simulink model "aircraft_sil"  (R2024a)
settings: Solver=ode45  StartTime=0.0  StopTime=2000  FixedStep=0.001  RelTol=1e-3
settings Model: PacingRate=100  Creator=ADMIN  LastModifiedBy=ADMIN

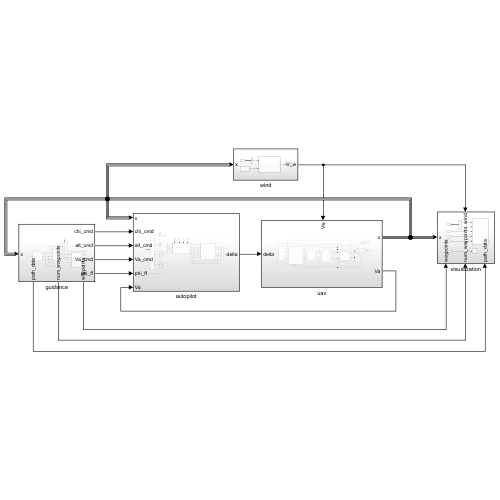
[thumbnail: Simulink's stored preview of the top-level diagram]
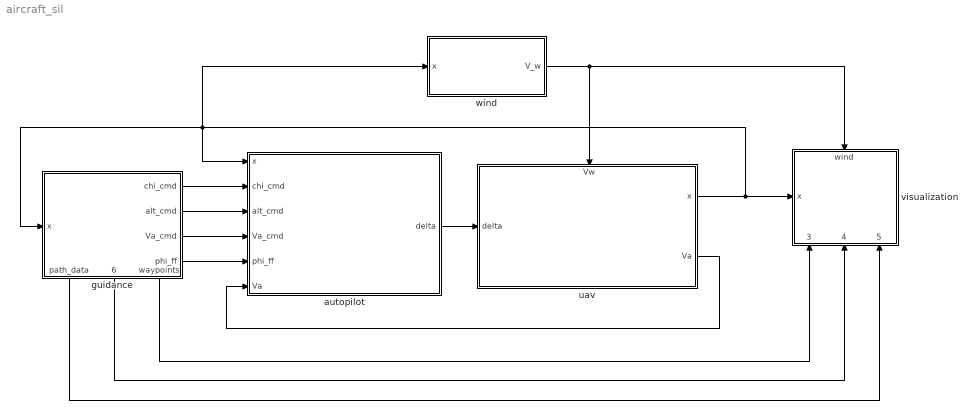
== system aircraft_sil ==
  "autopilot " : Subsystem
  guidance : Subsystem
      settings: PortSchema="{\"entries\":[{\"content\":{\"sides\":[{\"content\":{\"connectorIds\":[\"In1\"]},\"type\":\"ConnectorPlacement.EquallySpacedRectSide\",\"uuid\":\"7fb118f2-0b04-48cb-ae03-a27655c87a81\"},{\"content\":{\"connectorIds\":[\"Out1\",\"Out2\",\"Out3\",\"Out4\"],\"side\":\"RIGHT\"},\"type\":\"ConnectorPlacement.EquallySpacedRectSide\",\"uuid\":\"d962d9a4-ae5c-41e4-a82c-02c820f08147\"},{\"content\":{\"side\":\"TOP\"},\"type\":\"ConnectorPlacement.EquallySpacedRectSide\",\"uuid\":\"7cbabbb1-f237-4845-8a04-8eadc07c3469\"},{\"content\":{\"connectorIds\":[\"Out5\",\"Out6\",\"Out7\"],\"side\":\"BOTTOM\"},\"type\":\"ConnectorPlacement.EquallySpacedRectSide\",\"uuid\":\"34cfda24-2f18-4e48-95bb-4ae1da1686ef\"}]},\"type\":\"ConnectorPlacement.EquallySpacedConnector\",\"uuid\":\"2c187929-5ea7-462b-8474-1f36e513e0be\"}],\"packageUris\":[\"http://schema.mathworks.com/mf0/Connector/R2020b\"],\"version\":\"1.0\"}"
  "uav " : Subsystem
      settings: PortSchema="{\"entries\":[{\"content\":{\"sides\":[{\"content\":{\"connectorIds\":[\"In1\"]},\"type\":\"ConnectorPlacement.EquallySpacedRectSide\",\"uuid\":\"a7b46c76-63bb-4654-bcb2-91627cecb901\"},{\"content\":{\"connectorIds\":[\"Out1\",\"Out2\"],\"side\":\"RIGHT\"},\"type\":\"ConnectorPlacement.EquallySpacedRectSide\",\"uuid\":\"e45597e5-281a-43ae-9b8f-01f809ae90a8\"},{\"content\":{\"connectorIds\":[\"In2\"],\"side\":\"TOP\"},\"type\":\"ConnectorPlacement.EquallySpacedRectSide\",\"uuid\":\"e4f93d17-0834-49b6-953c-d959a9d487bc\"}]},\"type\":\"ConnectorPlacement.EquallySpacedConnector\",\"uuid\":\"aee35d44-0504-4876-b308-b0d63ae44a1f\"}],\"packageUris\":[\"http://schema.mathworks.com/mf0/Connector/R2020b\"],\"version\":\"1.0\"}"
  visualization : Subsystem
      settings: PortSchema="{\"entries\":[{\"content\":{\"sides\":[{\"content\":{\"connectorIds\":[\"In1\"]},\"type\":\"ConnectorPlacement.EquallySpacedRectSide\",\"uuid\":\"3ca85e6b-5690-4cee-b297-0410b8eb8b03\"},{\"content\":{\"side\":\"RIGHT\"},\"type\":\"ConnectorPlacement.EquallySpacedRectSide\",\"uuid\":\"b077d845-b4f0-4046-b1ae-a0ce879f315b\"},{\"content\":{\"connectorIds\":[\"In2\"],\"side\":\"TOP\"},\"type\":\"ConnectorPlacement.EquallySpacedRectSide\",\"uuid\":\"5282982d-07cb-4dd6-a7f3-d3fc714f27f8\"},{\"content\":{\"connectorIds\":[\"In3\",\"In4\",\"In5\"],\"side\":\"BOTTOM\"},\"type\":\"ConnectorPlacement.EquallySpacedRectSide\",\"uuid\":\"bf9b25fd-1836-4065-b749-44a2e35219bb\"}]},\"type\":\"ConnectorPlacement.EquallySpacedConnector\",\"uuid\":\"6eccf57b-fb72-419b-a501-32d6f52412a8\"}],\"packageUris\":[\"http://schema.mathworks.com/mf0/Connector/R2020b\"],\"version\":\"1.0\"}"
  wind : Subsystem
  wires:
  wind/1(V_w) -> visualization/2(wind), "uav "/2(Vw)
  "uav "/1(x) -> "autopilot "/1(x), guidance/1(x), wind/1(x), visualization/1(x)
  "autopilot "/1(delta) -> "uav "/1(delta)
  guidance/1(chi_cmd) -> "autopilot "/2(chi_cmd)
  guidance/2(alt_cmd) -> "autopilot "/3(alt_cmd)
  "uav "/2(Va) -> "autopilot "/6(Va)
  guidance/3(Va_cmd) -> "autopilot "/4(Va_cmd)
  guidance/4(phi_ff) -> "autopilot "/5(phi_ff)
  guidance/7(waypoints) -> visualization/3(waypoints)
  guidance/6(num_waypoints) -> visualization/4(num_waypoints)
  guidance/5(path_data) -> visualization/5(path_data)

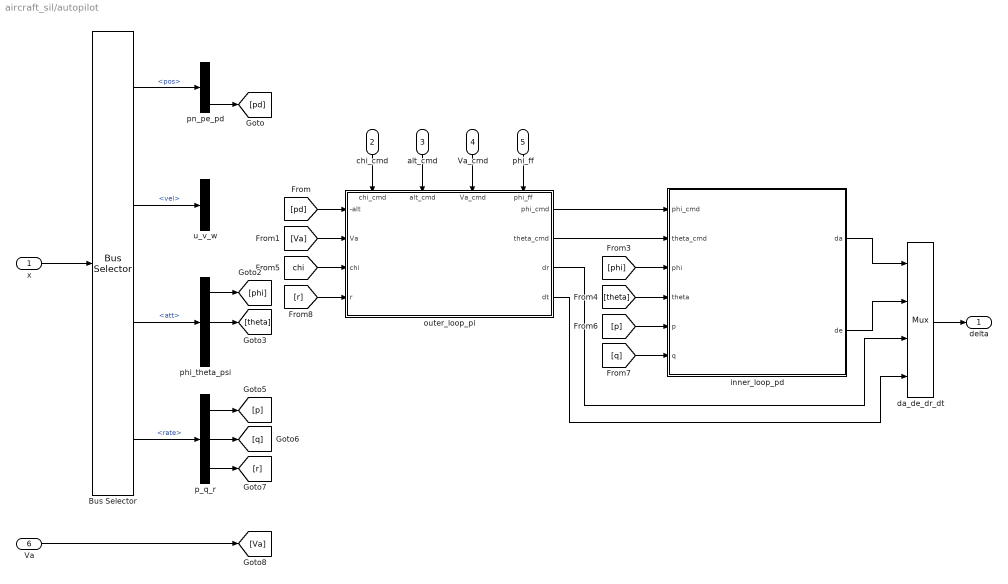
== system aircraft_sil/autopilot  ==
  x : Inport
  chi_cmd : Inport  Port=2
  alt_cmd : Inport  Port=3
  Va_cmd : Inport  Port=4
  phi_ff : Inport  Port=5
  Va : Inport  Port=6
  Bus Selector : BusSelector  OutputSignals=pos,vel,att,rate
  da_de_dr_dt : Mux
  inner_loop_pd : Subsystem
  outer_loop_pi : Subsystem
      settings: PortSchema="{\"entries\":[{\"content\":{\"sides\":[{\"content\":{\"connectorIds\":[\"In1\",\"In2\",\"In3\",\"In4\"]},\"type\":\"ConnectorPlacement.EquallySpacedRectSide\",\"uuid\":\"f8b93ce5-1209-4743-a4f6-40947377afa0\"},{\"content\":{\"connectorIds\":[\"Out1\",\"Out2\",\"Out3\",\"Out4\"],\"side\":\"RIGHT\"},\"type\":\"ConnectorPlacement.EquallySpacedRectSide\",\"uuid\":\"38b86da4-8ea0-4db2-a7be-1fc292de95ff\"},{\"content\":{\"connectorIds\":[\"In5\",\"In6\",\"In7\",\"In8\"],\"side\":\"TOP\"},\"type\":\"ConnectorPlacement.EquallySpacedRectSide\",\"uuid\":\"879dde49-1a12-4f2d-a7d9-4a8a8e5f8381\"}]},\"type\":\"ConnectorPlacement.EquallySpacedConnector\",\"uuid\":\"28f217f5-b437-4f7c-874d-3ab28b03532d\"}],\"packageUris\":[\"http://schema.mathworks.com/mf0/Connector/R2020b\"],\"version\":\"1.0\"}"
  p_q_r : Demux  Outputs=3
  phi_theta_psi : Demux  Outputs=3
  pn_pe_pd : Demux  Outputs=3
  u_v_w : Demux  Outputs=3
  delta : Outport
  wires:
  da_de_dr_dt/1 -> delta/1
  Bus Selector/3 -> phi_theta_psi/1  "<att>"
  Bus Selector/4 -> p_q_r/1  "<rate>"
  Bus Selector/1 -> pn_pe_pd/1  "<pos>"
  Bus Selector/2 -> u_v_w/1  "<vel>"
  inner_loop_pd/1(da) -> da_de_dr_dt/1
  inner_loop_pd/2(de) -> da_de_dr_dt/2
  outer_loop_pi/1(phi_cmd) -> inner_loop_pd/1(phi_cmd)
  outer_loop_pi/2(theta_cmd) -> inner_loop_pd/2(theta_cmd)
  outer_loop_pi/3(dr) -> da_de_dr_dt/3
  outer_loop_pi/4(dt) -> da_de_dr_dt/4
  pn_pe_pd/3 -> [pd]
  [pd] -> outer_loop_pi/1(-alt)
  [Va] -> outer_loop_pi/2(Va)
  phi_theta_psi/1 -> [phi]
  [phi] -> inner_loop_pd/3(phi)
  phi_theta_psi/2 -> [theta]
  [theta] -> inner_loop_pd/4(theta)
  [chi] -> outer_loop_pi/3(chi)
  p_q_r/1 -> [p]
  p_q_r/2 -> [q]
  [p] -> inner_loop_pd/5(p)
  [q] -> inner_loop_pd/6(q)
  p_q_r/3 -> [r]
  [r] -> outer_loop_pi/4(r)
  chi_cmd/1 -> outer_loop_pi/5(chi_cmd)
  alt_cmd/1 -> outer_loop_pi/6(alt_cmd)
  x/1 -> Bus Selector/1
  Va/1 -> [Va]
  Va_cmd/1 -> outer_loop_pi/7(Va_cmd)
  phi_ff/1 -> outer_loop_pi/8(phi_ff)

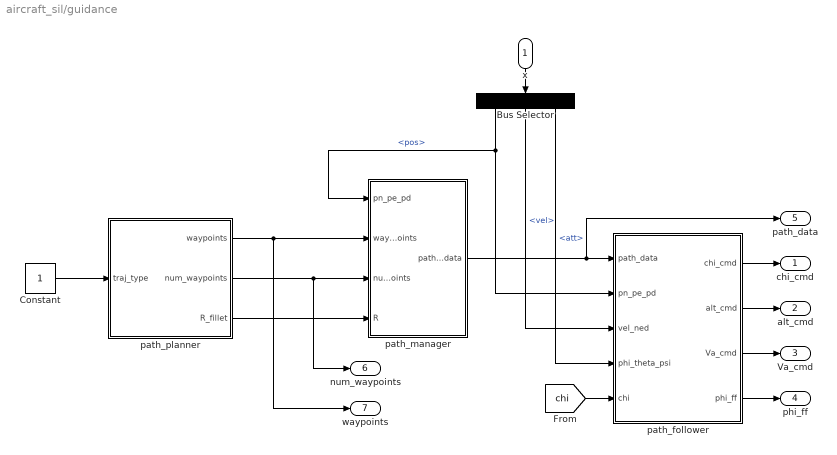
== system aircraft_sil/guidance ==
  x : Inport
  Bus Selector : BusSelector  OutputSignals=pos,vel,att
  Constant : Constant
  path_follower : MATLAB Function  TreatAsAtomicUnit=on
  path_manager : MATLAB Function  TreatAsAtomicUnit=on
  path_planner : MATLAB Function  TreatAsAtomicUnit=on
  chi_cmd : Outport
  alt_cmd : Outport  Port=2
  Va_cmd : Outport  Port=3
  phi_ff : Outport  Port=4
  path_data : Outport  Port=5
  num_waypoints : Outport  Port=6
  waypoints : Outport  Port=7
  wires:
  x/1 -> Bus Selector/1
  Bus Selector/1 -> path_manager/1(pn_pe_pd), path_follower/2(pn_pe_pd)  "<pos>"
  path_manager/1(path_data) -> path_data/1, path_follower/1(path_data)
  path_follower/1(chi_cmd) -> chi_cmd/1
  path_follower/2(alt_cmd) -> alt_cmd/1
  path_follower/3(Va_cmd) -> Va_cmd/1
  path_follower/4(phi_ff) -> phi_ff/1
  Bus Selector/2 -> path_follower/3(vel_ned)  "<vel>"
  Bus Selector/3 -> path_follower/4(phi_theta_psi)  "<att>"
  [chi] -> path_follower/5(chi)
  path_planner/1(waypoints) -> waypoints/1, path_manager/2(waypoints)
  path_planner/2(num_waypoints) -> num_waypoints/1, path_manager/3(num_waypoints)
  path_planner/3(R_fillet) -> path_manager/4(R)
  Constant/1 -> path_planner/1(traj_type)

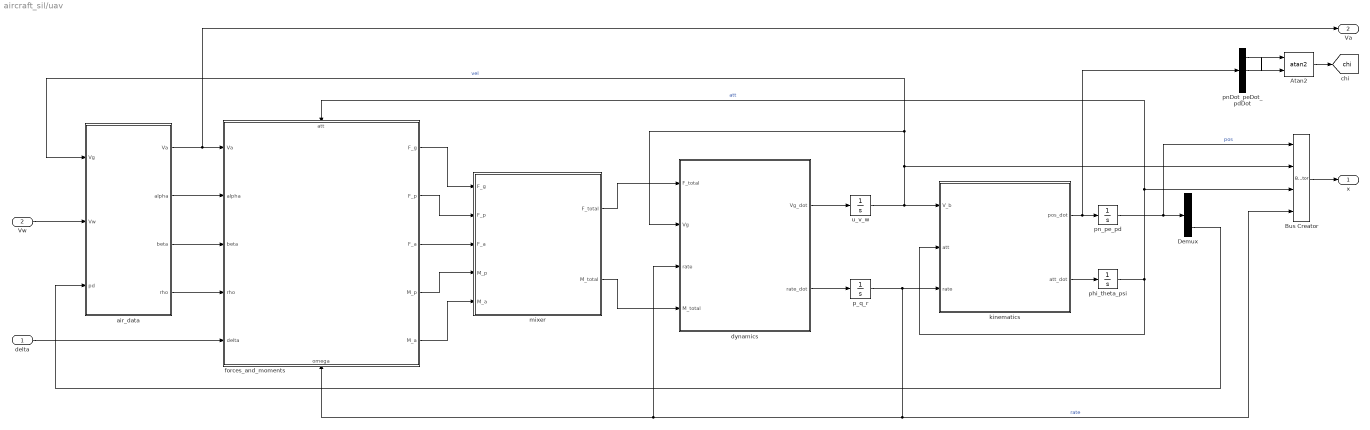
== system aircraft_sil/uav  ==
  delta : Inport
  Vw : Inport  Port=2
  Atan2 : Trigonometry  Operator=atan2
  Bus Creator : BusCreator  Inputs=4
  Demux : Demux  Outputs=3
  air_data : MATLAB Function  TreatAsAtomicUnit=on
  dynamics : Subsystem
  forces_and_moments : Subsystem
      settings: PortSchema="{\"entries\":[{\"content\":{\"sides\":[{\"content\":{\"connectorIds\":[\"In1\",\"In2\",\"In3\",\"In4\",\"In5\"]},\"type\":\"ConnectorPlacement.EquallySpacedRectSide\",\"uuid\":\"faed5ae1-1da7-4bdb-9f91-d07bb241893e\"},{\"content\":{\"connectorIds\":[\"Out1\",\"Out2\",\"Out3\",\"Out4\",\"Out5\"],\"side\":\"RIGHT\"},\"type\":\"ConnectorPlacement.EquallySpacedRectSide\",\"uuid\":\"3869cb38-1eed-4d47-9855-45677924a456\"},{\"content\":{\"connectorIds\":[\"In6\"],\"side\":\"TOP\"},\"type\":\"ConnectorPlacement.EquallySpacedRectSide\",\"uuid\":\"bdf63fef-403e-488a-a985-bca31845462f\"},{\"content\":{\"connectorIds\":[\"In7\"],\"side\":\"BOTTOM\"},\"type\":\"ConnectorPlacement.EquallySpacedRectSide\",\"uuid\":\"22a16173-6ad3-41e9-b567-c24186f01d1d\"}]},\"type\":\"ConnectorPlacement.EquallySpacedConnector\",\"uuid\":\"20fa0166-ef5c-40dd-8a30-826f9f2a65f7\"}],\"packageUris\":[\"http://schema.mathworks.com/mf0/Connector/R2020b\"],\"version\":\"1.0\"}"
  kinematics : Subsystem
  mixer : MATLAB Function  TreatAsAtomicUnit=on
  p_q_r : Integrator  InitialCondition=[0; 0; 0]
  phi_theta_psi : Integrator  InitialCondition=[0; 0.14622; 0]
  pnDot_peDot_pdDot : Demux  Outputs=3
  pn_pe_pd : Integrator  InitialCondition=[0; 0; -100]
  u_v_w : Integrator  InitialCondition=[15; 0; 3.3029]
  x : Outport
  Va : Outport  Port=2
  tag scope: chi=global
  wires:
  p_q_r/1 -> Bus Creator/4, dynamics/3(rate), forces_and_moments/7(omega), kinematics/3(rate)  "rate"
  kinematics/2(att_dot) -> phi_theta_psi/1
  u_v_w/1 -> kinematics/1(V_b), Bus Creator/2, air_data/1(Vg), dynamics/2(Vg)  "vel"
  pn_pe_pd/1 -> Bus Creator/1, Demux/1  "pos"
  dynamics/1(Vg_dot) -> u_v_w/1
  air_data/1(Va) -> Va/1, forces_and_moments/1(Va)
  phi_theta_psi/1 -> Bus Creator/3, forces_and_moments/6(att), kinematics/2(att)  "att"
  forces_and_moments/2(F_p) -> mixer/2(F_p)
  kinematics/1(pos_dot) -> pnDot_peDot_pdDot/1, pn_pe_pd/1
  forces_and_moments/3(F_a) -> mixer/3(F_a)
  Bus Creator/1 -> x/1
  mixer/1(F_total) -> dynamics/1(F_total)
  mixer/2(M_total) -> dynamics/4(M_total)
  Vw/1 -> air_data/2(Vw)
  air_data/2(alpha) -> forces_and_moments/2(alpha)
  air_data/3(beta) -> forces_and_moments/3(beta)
  forces_and_moments/1(F_g) -> mixer/1(F_g)
  forces_and_moments/4(M_p) -> mixer/4(M_p)
  air_data/4(rho) -> forces_and_moments/4(rho)
  forces_and_moments/5(M_a) -> mixer/5(M_a)
  Demux/3 -> air_data/3(pd)
  dynamics/2(rate_dot) -> p_q_r/1
  delta/1 -> forces_and_moments/5(delta)
  pnDot_peDot_pdDot/2 -> Atan2/1
  pnDot_peDot_pdDot/1 -> Atan2/2
  Atan2/1 -> [chi]

== system aircraft_sil/visualization ==
  x : Inport
  wind : Inport  Port=2
  waypoints : Inport  Port=3
  num_waypoints : Inport  Port=4
  path_data : Inport  Port=5
  Bus Selector : BusSelector  OutputSignals=pos,att
  MATLAB Function : MATLAB Function  TreatAsAtomicUnit=on
  wind_visualization : Scope
  wires:
  x/1 -> Bus Selector/1
  Bus Selector/1 -> MATLAB Function/1(pn_pe_pd)  "<pos>"
  Bus Selector/2 -> MATLAB Function/2(phi_theta_psi)  "<att>"
  wind/1 -> wind_visualization/1
  num_waypoints/1 -> MATLAB Function/4(num_waypoints)
  waypoints/1 -> MATLAB Function/3(waypoints)
  path_data/1 -> MATLAB Function/5(path_data)

== system aircraft_sil/wind ==
  x : Inport
  Bus Selector : BusSelector  OutputSignals=att
  Constant : Constant  Value=[0; 0; 0]
  MATLAB Function : MATLAB Function  TreatAsAtomicUnit=on
  V_w : Outport
  wires:
  x/1 -> Bus Selector/1
  Bus Selector/1 -> MATLAB Function/1(att)  "<att>"
  Constant/1 -> MATLAB Function/2(Vw_inertial)
  MATLAB Function/1(Vw) -> V_w/1

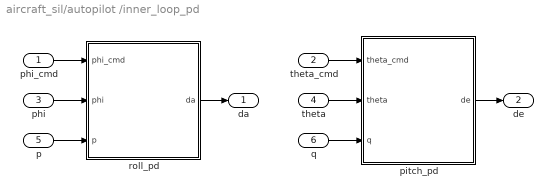
== system aircraft_sil/autopilot /inner_loop_pd ==
  phi_cmd : Inport
  theta_cmd : Inport  Port=2
  phi : Inport  Port=3
  theta : Inport  Port=4
  p : Inport  Port=5
  q : Inport  Port=6
  pitch_pd : Subsystem
  roll_pd : Subsystem
  da : Outport
  de : Outport  Port=2
  wires:
  phi/1 -> roll_pd/2(phi)
  theta_cmd/1 -> pitch_pd/1(theta_cmd)
  theta/1 -> pitch_pd/2(theta)
  q/1 -> pitch_pd/3(q)
  p/1 -> roll_pd/3(p)
  pitch_pd/1(de) -> de/1
  roll_pd/1(da) -> da/1
  phi_cmd/1 -> roll_pd/1(phi_cmd)

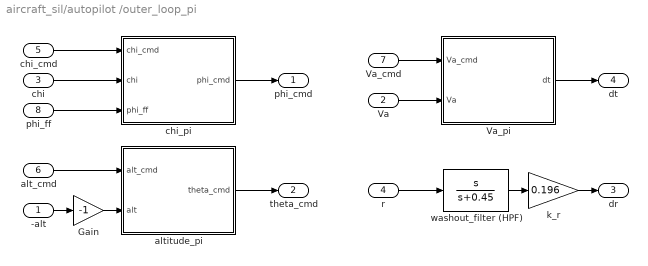
== system aircraft_sil/autopilot /outer_loop_pi ==
  -alt : Inport
  Va : Inport  Port=2
  chi : Inport  Port=3
  r : Inport  Port=4
  chi_cmd : Inport  Port=5
  alt_cmd : Inport  Port=6
  Va_cmd : Inport  Port=7
  phi_ff : Inport  Port=8
  Gain : Gain  Gain=-1
  Va_pi : Subsystem
  altitude_pi : Subsystem
  chi_pi : Subsystem
  k_r : Gain  Gain=0.196
  washout_filter (HPF) : TransferFcn  Numerator=[1 0]  Denominator=[1 0.45]
  phi_cmd : Outport
  theta_cmd : Outport  Port=2
  dr : Outport  Port=3
  dt : Outport  Port=4
  wires:
  Gain/1 -> altitude_pi/2(alt)
  -alt/1 -> Gain/1
  chi/1 -> chi_pi/2(chi)
  altitude_pi/1(theta_cmd) -> theta_cmd/1
  Va/1 -> Va_pi/2(Va)
  washout_filter (HPF)/1 -> k_r/1
  chi_pi/1(phi_cmd) -> phi_cmd/1
  Va_pi/1(dt) -> dt/1
  r/1 -> washout_filter (HPF)/1
  chi_cmd/1 -> chi_pi/1(chi_cmd)
  alt_cmd/1 -> altitude_pi/1(alt_cmd)
  k_r/1 -> dr/1
  Va_cmd/1 -> Va_pi/1(Va_cmd)
  phi_ff/1 -> chi_pi/3(phi_ff)

== system aircraft_sil/uav /dynamics ==
  F_total : Inport
  Vg : Inport  Port=2
  rate : Inport  Port=3
  M_total : Inport  Port=4
  rotational_dynamics : MATLAB Function  TreatAsAtomicUnit=on
  translational_dynamics : MATLAB Function  TreatAsAtomicUnit=on
  Vg_dot : Outport
  rate_dot : Outport  Port=2
  wires:
  rate/1 -> translational_dynamics/3(rate), rotational_dynamics/2(rate)
  M_total/1 -> rotational_dynamics/1(M_total)
  translational_dynamics/1(Vg_dot) -> Vg_dot/1
  rotational_dynamics/1(rate_dot) -> rate_dot/1
  Vg/1 -> translational_dynamics/2(Vg)
  F_total/1 -> translational_dynamics/1(F_total)

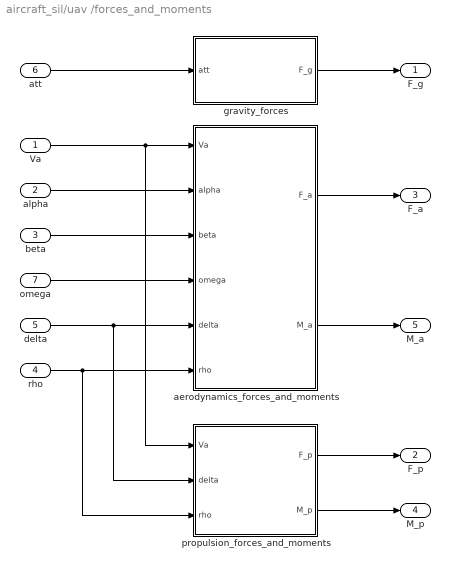
== system aircraft_sil/uav /forces_and_moments ==
  Va : Inport
  alpha : Inport  Port=2
  beta : Inport  Port=3
  rho : Inport  Port=4
  delta : Inport  Port=5
  att : Inport  Port=6
  omega : Inport  Port=7
  aerodynamics_forces_and_moments : MATLAB Function  TreatAsAtomicUnit=on
  gravity_forces : MATLAB Function  TreatAsAtomicUnit=on
  propulsion_forces_and_moments : MATLAB Function  TreatAsAtomicUnit=on
  F_g : Outport
  F_p : Outport  Port=2
  F_a : Outport  Port=3
  M_p : Outport  Port=4
  M_a : Outport  Port=5
  wires:
  beta/1 -> aerodynamics_forces_and_moments/3(beta)
  rho/1 -> propulsion_forces_and_moments/3(rho), aerodynamics_forces_and_moments/6(rho)
  att/1 -> gravity_forces/1(att)
  Va/1 -> propulsion_forces_and_moments/1(Va), aerodynamics_forces_and_moments/1(Va)
  alpha/1 -> aerodynamics_forces_and_moments/2(alpha)
  propulsion_forces_and_moments/1(F_p) -> F_p/1
  omega/1 -> aerodynamics_forces_and_moments/4(omega)
  propulsion_forces_and_moments/2(M_p) -> M_p/1
  aerodynamics_forces_and_moments/2(M_a) -> M_a/1
  aerodynamics_forces_and_moments/1(F_a) -> F_a/1
  gravity_forces/1(F_g) -> F_g/1
  delta/1 -> propulsion_forces_and_moments/2(delta), aerodynamics_forces_and_moments/5(delta)

== system aircraft_sil/uav /kinematics ==
  V_b : Inport
  att : Inport  Port=2
  rate : Inport  Port=3
  rotational_kinematics : MATLAB Function  TreatAsAtomicUnit=on
  translational_kinematics : MATLAB Function  TreatAsAtomicUnit=on
  pos_dot : Outport
  att_dot : Outport  Port=2
  wires:
  translational_kinematics/1(pos_dot) -> pos_dot/1
  rate/1 -> rotational_kinematics/1(rate)
  att/1 -> rotational_kinematics/2(att), translational_kinematics/2(att)
  rotational_kinematics/1(att_dot) -> att_dot/1
  V_b/1 -> translational_kinematics/1(V_b)

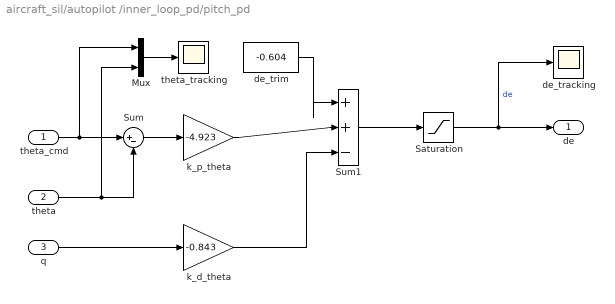
== system aircraft_sil/autopilot /inner_loop_pd/pitch_pd ==
  theta_cmd : Inport
  theta : Inport  Port=2
  q : Inport  Port=3
  Mux : Mux  Inputs=2
  Saturation : Saturate  UpperLimit=1  LowerLimit=-1
  Sum : Sum  Inputs=|+-
  Sum1 : Sum  Inputs=|++-
  de_tracking : Scope
  de_trim : Constant  Value=-0.604
  k_d_theta : Gain  Gain=-0.843
  k_p_theta : Gain  Gain=-4.923
  theta_tracking : Scope
  de : Outport
  wires:
  Saturation/1 -> de/1, de_tracking/1  "de"
  Sum1/1 -> Saturation/1
  q/1 -> k_d_theta/1
  Sum/1 -> k_p_theta/1
  theta_cmd/1 -> Mux/1, Sum/1
  theta/1 -> Mux/2, Sum/2
  Mux/1 -> theta_tracking/1
  k_p_theta/1 -> Sum1/2
  k_d_theta/1 -> Sum1/3
  de_trim/1 -> Sum1/1

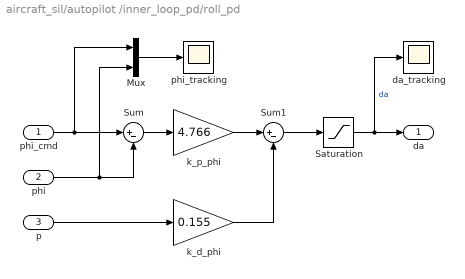
== system aircraft_sil/autopilot /inner_loop_pd/roll_pd ==
  phi_cmd : Inport
  phi : Inport  Port=2
  p : Inport  Port=3
  Mux : Mux  Inputs=2
  Saturation : Saturate  UpperLimit=0.436  LowerLimit=-0.436
  Sum : Sum  Inputs=|+-
  Sum1 : Sum  Inputs=|+-
  da_tracking : Scope
  k_d_phi : Gain  Gain=0.155
  k_p_phi : Gain  Gain=4.766
  phi_tracking : Scope
  da : Outport
  wires:
  k_d_phi/1 -> Sum1/2
  phi/1 -> Sum/2, Mux/2
  Sum/1 -> k_p_phi/1
  p/1 -> k_d_phi/1
  phi_cmd/1 -> Mux/1, Sum/1
  Sum1/1 -> Saturation/1
  Saturation/1 -> da_tracking/1, da/1  "da"
  Mux/1 -> phi_tracking/1
  k_p_phi/1 -> Sum1/1

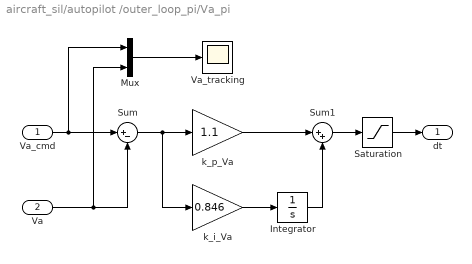
== system aircraft_sil/autopilot /outer_loop_pi/Va_pi ==
  Va_cmd : Inport
  Va : Inport  Port=2
  Integrator : Integrator  LimitOutput=on  UpperSaturationLimit=1  LowerSaturationLimit=0
  Mux : Mux  Inputs=2
  Saturation : Saturate  UpperLimit=1  LowerLimit=0
  Sum : Sum  Inputs=|+-
  Sum1 : Sum  Inputs=|++
  Va_tracking : Scope
  k_i_Va : Gain  Gain=0.846
  k_p_Va : Gain  Gain=1.1
  dt : Outport
  wires:
  k_p_Va/1 -> Sum1/1
  Mux/1 -> Va_tracking/1
  Saturation/1 -> dt/1
  Sum1/1 -> Saturation/1
  Va_cmd/1 -> Sum/1, Mux/1
  Sum/1 -> k_i_Va/1, k_p_Va/1
  Va/1 -> Sum/2, Mux/2
  k_i_Va/1 -> Integrator/1
  Integrator/1 -> Sum1/2

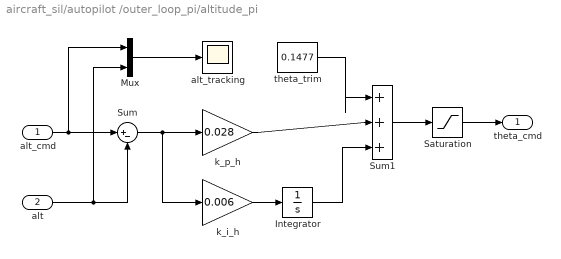
== system aircraft_sil/autopilot /outer_loop_pi/altitude_pi ==
  alt_cmd : Inport
  alt : Inport  Port=2
  Integrator : Integrator  LimitOutput=on  UpperSaturationLimit=0.261  LowerSaturationLimit=-0.261
  Mux : Mux  Inputs=2
  Saturation : Saturate  UpperLimit=0.9  LowerLimit=-0.9
  Sum : Sum  Inputs=|+-
  Sum1 : Sum  Inputs=|+++
  alt_tracking : Scope
  k_i_h : Gain  Gain=0.006
  k_p_h : Gain  Gain=0.028
  theta_trim : Constant  Value=0.1477
  theta_cmd : Outport
  wires:
  Mux/1 -> alt_tracking/1
  Saturation/1 -> theta_cmd/1
  Sum1/1 -> Saturation/1
  alt_cmd/1 -> Sum/1, Mux/1
  Sum/1 -> k_i_h/1, k_p_h/1
  alt/1 -> Mux/2, Sum/2
  k_i_h/1 -> Integrator/1
  Integrator/1 -> Sum1/3
  k_p_h/1 -> Sum1/2
  theta_trim/1 -> Sum1/1

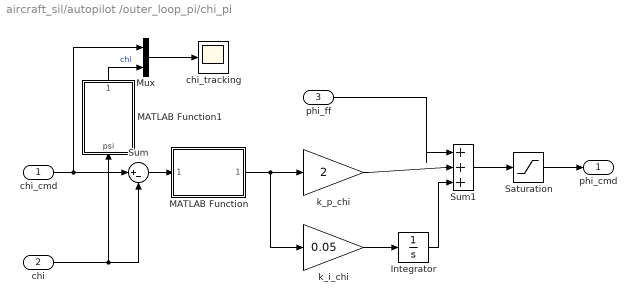
== system aircraft_sil/autopilot /outer_loop_pi/chi_pi ==
  chi_cmd : Inport
  chi : Inport  Port=2
  phi_ff : Inport  Port=3
  Integrator : Integrator  LimitOutput=on  UpperSaturationLimit=0.436  LowerSaturationLimit=-0.436
  MATLAB Function : MATLAB Function  TreatAsAtomicUnit=on
  MATLAB Function1 : MATLAB Function  TreatAsAtomicUnit=on
  Mux : Mux  Inputs=2
  Saturation : Saturate  UpperLimit=0.436  LowerLimit=-0.436
  Sum : Sum  Inputs=|+-
  Sum1 : Sum  Inputs=|+++
  chi_tracking : Scope
  k_i_chi : Gain  Gain=0.05
  k_p_chi : Gain  Gain=2
  phi_cmd : Outport
  wires:
  Integrator/1 -> Sum1/3
  k_i_chi/1 -> Integrator/1
  chi/1 -> Sum/2, MATLAB Function1/1(psi)
  Sum/1 -> MATLAB Function/1(error_in)
  Sum1/1 -> Saturation/1
  Saturation/1 -> phi_cmd/1
  Mux/1 -> chi_tracking/1
  k_p_chi/1 -> Sum1/2
  MATLAB Function/1(error_out) -> k_i_chi/1, k_p_chi/1
  chi_cmd/1 -> Mux/1, Sum/1
  MATLAB Function1/1(psi_wrapped) -> Mux/2  "chi"
  phi_ff/1 -> Sum1/1

== matlab function aircraft_sil/uav /kinematics/rotational_kinematics ==
  data: rate input; att_dot output size=[3, 1]; att input
function att_dot = rot_kinematics(rate, att)
    % inputs:
    %   rate:   [3x1] angular rates [p; q; r] (rad/s)
    %   att:     [3x1] euler angles [phi; theta; psi] (rad)
    % outputs:
    %   att_dot: [3x1] euler angle derivatives [phi_dot; theta_dot; psi_dot] (rad/s)

    p = rate(1); q = rate(2); r = rate(3);
    phi = att(1); theta = att(2);

    cphi = cos(phi); sphi = sin(phi);
    cthe = cos(theta); tthe = tan(theta);

    R_rot = [1, sphi*tthe, cphi*tthe;
             0, cphi,      -sphi;
             0, sphi/cthe, cphi/cthe];
             
    att_dot = R_rot * [p; q; r];
end

== matlab function aircraft_sil/uav /kinematics/translational_kinematics ==
  data: V_b input; pos_dot output size=[3, 1]; att input
function pos_dot = trans_kinematics(V_b, att)
    % inputs:
    %   V_b:     [3x1] body velocities [u; v; w] (m/s)
    %   att:     [3x1] euler angles [phi; theta; psi] (rad)
    % outputs:
    %   pos_dot: [3x1] inertial pos derivatives [pn_dot; pe_dot; pd_dot] (m/s)

    u = V_b(1); v = V_b(2); w = V_b(3);
    phi = att(1); theta = att(2); psi = att(3);

    cphi = cos(phi); sphi = sin(phi);
    cthe = cos(theta); sthe = sin(theta);
    cpsi = cos(psi); spsi = sin(psi);

    R_b_v = [cthe*cpsi, sphi*sthe*cpsi - cphi*spsi, cphi*sthe*cpsi + sphi*spsi;
             cthe*spsi, sphi*sthe*spsi + cphi*cpsi, cphi*sthe*spsi - sphi*cpsi;
             -sthe,     sphi*cthe,                  cphi*cthe];
             
    pos_dot = R_b_v * [u; v; w];
end

== matlab function aircraft_sil/autopilot /outer_loop_pi/chi_pi/MATLAB Function ==
  data: error_in input; error_out output
function error_out = wrap_angle(error_in)
    % wrap angle to [-pi, pi]
    error_out = mod(error_in + pi, 2*pi) - pi;
end

== matlab function aircraft_sil/visualization/MATLAB Function ==
  data: pn_pe_pd input; phi_theta_psi input; waypoints input; num_waypoints input; path_data input
function draw_uav_3d(pn_pe_pd, phi_theta_psi, waypoints, num_waypoints, path_data)
    coder.extrinsic('update_uav_plot');
    update_uav_plot(pn_pe_pd, phi_theta_psi, waypoints, num_waypoints, path_data);
end

== matlab function aircraft_sil/guidance/path_manager ==
  settings: updateMethod=DISCRETE  sampleTime=0.02
  data: pn_pe_pd input size=[3,1]; path_data output size=[12, 1]; waypoints input; num_waypoints input; R input
function path_data = path_manager(pn_pe_pd, waypoints, num_waypoints, R)
    % persistent state machine variables
    persistent state ptr_a
    if isempty(state)
        state = 1;  % 1 = line, 2 = fillet orbit
        ptr_a = 1;
    end

    p = pn_pe_pd;

    % wrap waypoint indices
    idx_a = ptr_a;
    idx_b = mod(ptr_a, num_waypoints) + 1;
    idx_c = mod(ptr_a + 1, num_waypoints) + 1;

    % active waypoint coordinates
    w_a = waypoints(idx_a, :)';
    w_b = waypoints(idx_b, :)';
    w_c = waypoints(idx_c, :)';

    % path direction vectors
    q_prev = (w_b - w_a) / norm(w_b - w_a);
    q_next = (w_c - w_b) / norm(w_c - w_b);

    % fillet geometry
    rho      = acos(-q_prev' * q_next);
    d_fillet = R / tan(rho / 2);

    % state machine
    switch state
        case 1  % straight line
            z = w_b - d_fillet * q_prev;

            % check if UAV crossed the half-plane
            if (p - z)' * q_prev > 0
                state = 2;
            end

        case 2  % orbit
            z = w_b + d_fillet * q_next;

            % check if UAV crossed the half-plane
            if (p - z)' * q_next > 0
                state = 1;
                ptr_a = mod(ptr_a, num_waypoints) + 1;
            end
    end

    % initialize outputs
    flag = 0;
    c_n = 0;  c_e = 0;  c_d = 0;
    r_n = 0;  r_e = 0;  r_d = 0;
    q_n = 1;  q_e = 0;  q_d = 0;
    lambda = 1;

    % define active path
    switch state
        case 1  % line
            r_n = w_a(1);  r_e = w_a(2);  r_d = w_a(3);
            q_n = q_prev(1);  q_e = q_prev(2);  q_d = q_prev(3);

        case 2  % orbit
            flag = 1;

            q_diff = q_prev - q_next;
            c = w_b - (R / sin(rho / 2)) * q_diff / norm(q_diff);

            c_n = c(1);  c_e = c(2);  c_d = c(3);
            lambda = sign(q_prev(1) * q_next(2) - ...
                          q_prev(2) * q_next(1));
    end

    path_data = [flag; c_n; c_e; c_d; R; lambda; ...
                 r_n; r_e; r_d; q_n; q_e; q_d];
end

== matlab function aircraft_sil/wind/MATLAB Function ==
  data: att input; Vw output; Vw_inertial input
function Vw = rotate_wind(att, Vw_inertial)
    phi     = att(1);
    theta   = att(2);
    psi     = att(3);

    % rotation matrix from inertial to body frame (R_v^b)
    R_yaw   = [  cos(psi),  sin(psi),           0;
                -sin(psi),  cos(psi),           0;
                        0,         0,          1];
    R_pitch = [cos(theta),         0, -sin(theta);
                        0,         1,           0;
               sin(theta),         0, cos(theta)];
    R_roll  = [         1,         0,           0;
                        0,  cos(phi),    sin(phi);
                        0, -sin(phi),   cos(phi)];
    
    R_v_to_b = R_roll * R_pitch * R_yaw;
    
    % total body frame wind (ready for gusts to be added later)
    Vw = R_v_to_b * Vw_inertial;
end

== matlab function aircraft_sil/autopilot /outer_loop_pi/chi_pi/MATLAB Function1 ==
  data: psi input; psi_wrapped output
function psi_wrapped = wrap_plot(psi)
    psi_wrapped = mod(psi + pi, 2*pi) - pi;
end

== matlab function aircraft_sil/guidance/path_follower ==
  settings: updateMethod=DISCRETE  sampleTime=0.02
  data: path_data input size=[12,1]; pn_pe_pd input size=[3,1]; chi_cmd output size=[1, 1]; alt_cmd output; Va_cmd output; phi_ff output; vel_ned input size=[3,1]; phi_theta_psi input size=[3,1]; chi input size=[1,1]
function [chi_cmd, alt_cmd, Va_cmd, phi_ff] = ...
    path_follower(path_data, pn_pe_pd, vel_ned, phi_theta_psi, chi)

%% initialize commands and parameters
    Va_cmd = 15.0;

    k_orbit = 3.0;
    k_path  = 0.05;
    chi_inf = pi / 2;
    gravity = 9.81;

%% unpack path data
    flag   = path_data(1);
    c_n    = path_data(2);   c_e    = path_data(3);   c_d    = path_data(4);
    R      = path_data(5);   lambda = path_data(6);
    r_n    = path_data(7);   r_e    = path_data(8);   r_d    = path_data(9);
    q_n    = path_data(10);  q_e    = path_data(11);  q_d    = path_data(12);

%% extract states
    pn = pn_pe_pd(1);
    pe = pn_pe_pd(2);

    psi     = phi_theta_psi(3);
    chi_val = chi(1);

    % extract horizontal ground speed magnitude
    Vg = sqrt(vel_ned(1)^2 + vel_ned(2)^2);

%% path following logic
    if flag == 1

        % orbit vector field
        d     = sqrt((pn - c_n)^2 + (pe - c_e)^2);
        varphi = atan2(pe - c_e, pn - c_n);

        % wrap phase error to [-pi, pi]
        while (varphi - chi_val) < -pi
            varphi = varphi + 2 * pi;
        end

        while (varphi - chi_val) > pi
            varphi = varphi - 2 * pi;
        end

        % course command
        chi_cmd = varphi + lambda * ...
            (pi / 2 + atan(k_orbit * (d - R) / R));

        alt_cmd = -c_d;

        % feedforward roll command
        if Vg < 0.1
            phi_ff = 0.0;
        else
            phi_ff = lambda * atan( ...
                Vg^2 / (R * gravity * cos(chi_val - psi)));
        end

    else

        % straight-line vector field
        chi_q = atan2(q_e, q_n);

        % wrap course error to [-pi, pi]
        while (chi_q - chi_val) < -pi
            chi_q = chi_q + 2 * pi;
        end

        while (chi_q - chi_val) > pi
            chi_q = chi_q - 2 * pi;
        end

        % cross-track error
        e_py = -sin(chi_q) * (pn - r_n) + ...
                cos(chi_q) * (pe - r_e);

        % course command
        chi_cmd = chi_q - chi_inf * (2 / pi) * atan(k_path * e_py);

        % dynamic altitude command
        s_n     = pn - r_n;
        s_e     = pe - r_e;
        q_mag_h = sqrt(q_n^2 + q_e^2);

        if q_mag_h == 0
            alt_cmd = -r_d;
        else
            alt_cmd = -r_d - ...
                sqrt(s_n^2 + s_e^2) * q_d / q_mag_h;
        end

        % wings level for straight-line paths
        phi_ff = 0.0;
    end
end

== matlab function aircraft_sil/guidance/path_planner ==
  settings: updateMethod=DISCRETE  sampleTime=0.02
  data: traj_type input size=1; waypoints output size=[100, 3]; num_waypoints output size=1; R_fillet output size=1
function [waypoints, num_waypoints, R_fillet] = path_planner(traj_type)
    % preallocate maximum array size to prevent simulink dimension errors
    MAX_WP = 100;
    waypoints = zeros(MAX_WP, 3);
    
    % default fallback variables
    num_waypoints = 1;
    R_fillet = 50; 

    switch traj_type
        case 1 % 3d ascending star
            num_waypoints = 40;
            R_fillet = 80;
            for i = 1:num_waypoints
                if mod(i, 2) == 0, r = 1000; else, r = 400; end
                angle = (i-1) * (2*pi / 10);
                waypoints(i, :) = [r*cos(angle), r*sin(angle), -100 - i*15];
            end
            
        case 2 % tight lawnmower
            num_waypoints = 10;
            R_fillet = 35;
            for i = 1:25
                waypoints(4*i-3, :) = [0, (i-1)*160, -100];
                waypoints(4*i-2, :) = [500, (i-1)*160, -100];
                waypoints(4*i-1, :) = [500, (i-1)*160 + 80, -100];
                waypoints(4*i, :)   = [0, (i-1)*160 + 80, -100];
            end
    end
end

== matlab function aircraft_sil/uav /forces_and_moments/gravity_forces ==
  data: att input; F_g output; P parameter
function F_g = calculate_gravity(att, P)
    % inputs:
    %   att:  [3x1] euler angles [phi; theta; psi] (rad)
    %   mass: [1x1] uav mass (kg)
    %   g:    [1x1] gravitational constant (m/s^2)
    % outputs:
    %   F_g:  [3x1] gravity forces [fx; fy; fz] (n)
    
    phi   = att(1);
    theta = att(2);
    
    % project gravity to body frame
    F_g = P.mass * P.g * [-sin(theta);
                           cos(theta) * sin(phi);
                           cos(theta) * cos(phi)];
end

== matlab function aircraft_sil/uav /air_data ==
  data: Vg input; Va output; Vw input; pd input; alpha output; beta output; rho output; P parameter
function [Va, alpha, beta, rho] = calculate_env_data(Vg, Vw, pd, P)
    % inputs:
    %   Vg: [3x1] body-frame ground velocity [u; v; w] (m/s)
    %   Vw: [3x1] body-frame wind velocity [uw; vw; ww] (m/s)
    %   pd:  [1x1] down position (negative of altitude) (m)
    % outputs:
    %   Va:     [1x1] airspeed magnitude (m/s)
    %   alpha:  [1x1] angle of attack (rad)
    %   beta:   [1x1] sideslip angle (rad)
    
    % current height
    h = -pd;
    
    % temperature and pressure at altitude h
    T = P.T0 + P.L0 * h;
    p = P.p0 * (P.T0 / T)^((P.g * P.Molar) / (P.R * P.L0));
    
    % dynamic density using ideal gas law
    rho = (p * P.Molar) / (P.R * T);
    
    % airspeed vector
    V_r = Vg - Vw;
    
    % airspeed magnitude
    Va = norm(V_r);
    
    % angle of attack and sideslip
    if Va == 0 % prevent to divide by zero
        alpha = 0;
        beta  = 0;
    else
        alpha = atan2(V_r(3), V_r(1));
        beta  = asin(V_r(2) / Va);
    end
end

== matlab function aircraft_sil/uav /forces_and_moments/aerodynamics_forces_and_moments ==
  data: Va input; F_a output; alpha input; beta input; M_a output; omega input; delta input size=[4, 1]; rho input; P parameter
function [F_a, M_a] = calculate_aerodynamics(Va, alpha, beta, ...
                                             omega, delta, rho, P)
    % inputs:
    %   Va:    [1x1] airspeed (m/s)
    %   alpha: [1x1] angle of attack (rad)
    %   beta:  [1x1] sideslip angle (rad)
    %   omega: [3x1] body angular rates [p; q; r] (rad/s)
    %   delta: [4x1] control signals [da; de; dr; dt]
    %   rho:   [1x1] air density (kg/m^3)
    %   P:     [1x1 struct] aerodynamic parameters
    % outputs:
    %   F_a:   [3x1] aerodynamic forces [fax; fay; faz] (n)
    %   M_a:   [3x1] aerodynamic moments [max; may; maz] (n-m)
    
    p = omega(1);
    q = omega(2);
    r = omega(3);
    
    da = delta(1);
    de = delta(2);
    dr = delta(3);
    
    % prevent division by zero at rest
    if Va == 0
        F_a = [0; 0; 0];
        M_a = [0; 0; 0];
        return;
    end
    
    % sigmoid blending function for non-linear stall
    sig_num = 1 + exp(-P.M * (alpha - P.alpha0)) + ...
        exp(P.M * (alpha + P.alpha0));
    sig_den = (1 + exp(-P.M * (alpha - P.alpha0))) * ...
        (1 + exp(P.M * (alpha + P.alpha0)));
    sigma_alpha = sig_num / sig_den;
    
    % non-linear lift coefficient
    CL_linear = P.C_L0 + P.C_Lalpha * alpha;
    CL_flat   = 2 * sign(alpha) * sin(alpha)^2 * cos(alpha);
    CL_alpha  = (1 - sigma_alpha) * CL_linear + sigma_alpha * CL_flat;
    
    % non-linear drag coefficient (quadratic)
    AR = (P.b^2) / P.S;
    CD_alpha = P.C_D0 + (CL_linear^2) / (pi * P.e * AR);
    
    % longitudinal aerodynamic coefficients
    cx      = -CD_alpha * cos(alpha) + CL_alpha * sin(alpha);
    cx_q    = -P.C_Dq * cos(alpha) + P.C_Lq * sin(alpha);
    cx_de   = -P.C_Dde * cos(alpha) + P.C_Lde * sin(alpha);
    
    cz      = -CD_alpha * sin(alpha) - CL_alpha * cos(alpha);
    cz_q    = -P.C_Dq * sin(alpha) - P.C_Lq * cos(alpha);
    cz_de   = -P.C_Dde * sin(alpha) - P.C_Lde * cos(alpha);
    
    % dynamic pressure terms
    q_bar = 0.5 * rho * Va^2 * P.S;
    c_2v  = (P.c * q) / (2 * Va);
    b_2v_p = (P.b * p) / (2 * Va);
    b_2v_r = (P.b * r) / (2 * Va);
    
    % compute forces
    fax = q_bar * (cx + cx_q * c_2v + cx_de * de);
    fay = q_bar * (P.C_Y0 + P.C_Ybeta * beta + P.C_Yp * b_2v_p + ...
        P.C_Yr * b_2v_r + P.C_Yda * da + P.C_Ydr * dr);
    faz = q_bar * (cz + cz_q * c_2v + cz_de * de);
    
    % compute moments
    max = q_bar * P.b * (P.C_Mx0 + P.C_Mxbeta * beta + ...
        P.C_Mxp * b_2v_p + P.C_Mxr * b_2v_r + ...
        P.C_Mxda * da + P.C_Mxdr * dr);
    may = q_bar * P.c * (P.C_My0 + P.C_Myalpha * alpha + ...
        P.C_Myq * c_2v + P.C_Myde * de);
    maz = q_bar * P.b * (P.C_Mz0 + P.C_Mzbeta * beta + ...
        P.C_Mzp * b_2v_p + P.C_Mzr * b_2v_r + ...
        P.C_Mzda * da + P.C_Mzdr * dr);
    
    F_a = [fax; fay; faz];
    M_a = [max; may; maz];
end

== matlab function aircraft_sil/uav /forces_and_moments/propulsion_forces_and_moments ==
  data: Va input; F_p output; delta input; M_p output; rho input; P parameter
function [F_p, M_p] = calculate_propulsion(Va, delta, rho, P)
    % calculates propulsion forces and moments[cite: 1]
    % inputs:
    %   Va:   [1x1] airspeed (m/s)
    %   delta:[4x1] control signals [da; de; dr; dt]
    %   rho:  [1x1] air density (kg/m^3)
    %   P:    [1x1 struct] physical parameters
    % outputs:
    %   F_p:  [3x1] propulsive force [fx; fy; fz] (n)
    %   M_p:  [3x1] propulsive moment [mx; my; mz] (n-m)

    dt = delta(4);
    if dt == 0
        F_p = [0; 0; 0];
        M_p = [0; 0; 0];
        return;
    end
    
    v_in = P.V_max * dt;
    
    a = (rho * P.D_prop^5) / ((2 * pi)^2) * P.C_Q0;
    b = (rho * P.D_prop^4) / (2 * pi) * P.C_Q1 * Va + ...
        (P.k_Q * P.k_V) / P.R_motor;
    c = rho * P.D_prop^3 * P.C_Q2 * Va^2 - ...
        (P.k_Q / P.R_motor) * v_in + P.k_Q * P.i0;
    
    omega_p = (-b + sqrt(b^2 - 4 * a * c)) / (2 * a);
    
    t_p = (rho * P.D_prop^4) / ((2 * pi)^2) * omega_p^2 * P.C_T0 + ...
          (rho * P.D_prop^3) / (2 * pi) * omega_p * Va * P.C_T1 + ...
          rho * P.D_prop^2 * Va^2 * P.C_T2;
          
    q_p = (rho * P.D_prop^5) / ((2 * pi)^2) * omega_p^2 * P.C_Q0 + ...
          (rho * P.D_prop^4) / (2 * pi) * omega_p * Va * P.C_Q1 + ...
          rho * P.D_prop^3 * Va^2 * P.C_Q2;
          
    F_p = [t_p; 0; 0];
    M_p = [-q_p; 0; 0];
end

== matlab function aircraft_sil/uav /mixer ==
  data: F_g input; F_total output; F_p input; F_a input; M_p input; M_a input; M_total output
function [F_total, M_total] = mix_forces_moments(F_g, F_p, F_a, M_p, M_a)
    % sums all forces and moments[cite: 1]
    % inputs:
    %   F_g: [3x1] gravity force (n)
    %   F_p: [3x1] propulsive force (n)
    %   F_a: [3x1] aerodynamic force (n)
    %   M_p: [3x1] propulsive moment (n-m)
    %   M_a: [3x1] aerodynamic moment (n-m)
    % outputs:
    %   F_total: [3x1] total body frame force (n)
    %   M_total: [3x1] total body frame moment (n-m)

    F_total = F_g + F_p + F_a;
    M_total = M_p + M_a;
end

== matlab function aircraft_sil/uav /dynamics/translational_dynamics ==
  data: F_total input; Vg input; Vg_dot output size=[3, 1]; rate input; P parameter
function Vg_dot = trans_dynamics(F_total, Vg, rate, P)
    % inputs:
    %   F_total: [3x1] total forces [fx; fy; fz] (n)
    %   Vg:     [3x1] body velocities [u; v; w] (m/s)
    %   rate:   [3x1] angular rates [p; q; r] (rad/s)
    %   P:       [1x1 struct] physical parameters
    % outputs:
    %   Vg_dot: [3x1] velocity derivatives [u_dot; v_dot; w_dot] (m/s^2)

    u = Vg(1); v = Vg(2); w = Vg(3);
    p = rate(1); q = rate(2); r = rate(3);
    fx = F_total(1); 
    fy = F_total(2); 
    fz = F_total(3);

    u_dot = r*v - q*w + fx / P.mass;
    v_dot = p*w - r*u + fy / P.mass;
    w_dot = q*u - p*v + fz / P.mass;
    
    Vg_dot = [u_dot; v_dot; w_dot];
end

== matlab function aircraft_sil/uav /dynamics/rotational_dynamics ==
  data: M_total input; rate_dot output size=[3, 1]; rate input; P parameter
function rate_dot = rot_dynamics(M_total, rate, P)
    % inputs:
    %   M_total:   [3x1] total moments [mx; my; mz] (n-m)
    %   rate:     [3x1] angular rates [p; q; r] (rad/s)
    %   P:         [1x1 struct] physical parameters
    % outputs:
    %   rate_dot: [3x1] angular rate derivatives [p_dot; q_dot; r_dot] (rad/s^2)

    p = rate(1); q = rate(2); r = rate(3);
    mx = M_total(1); my = M_total(2); mz = M_total(3);

    p_dot = P.Gamma1*p*q - P.Gamma2*q*r + P.Gamma3*mx + P.Gamma4*mz;
    q_dot = P.Gamma5*p*r - P.Gamma6*(p^2 - r^2) + my / P.Jy;
    r_dot = P.Gamma7*p*q - P.Gamma1*q*r + P.Gamma4*mx + P.Gamma8*mz;
    
    rate_dot = [p_dot; q_dot; r_dot];
end
